simulink model "Identyfikacja"  (R2015a)
settings: Solver=ode4  StartTime=0.0  StopTime=tSim  FixedStep=0.01  RelTol=1e-3
values from neighbouring files (symbols this model uses):
  c1 = Parametry(1)    [skryptDoIdentyfikacji.m]    (also in wskaznikJakosci.m = params(1))
  c2 = Parametry(2)    [skryptDoIdentyfikacji.m]    (also in wskaznikJakosci.m = params(2))
  c3 = Parametry(3)    [skryptDoIdentyfikacji.m]    (also in wskaznikJakosci.m = params(3))
  p1 = polyfit(PWM_level, pred_napelniania, 2)    [chka_zawor_gora.m]    (also in skryptDoIdentyfikacji.m = [-49.142857142857010 99.114285714285490 -23.369999999999905]; wskaznikJakosci.m = [-49.142857142857010 99.114285714285490 -23.369999999999905])
  PWM = 0.4    [chka_zawor_gora.m]    (also in skryptDoIdentyfikacji.m = 1; wskaznikJakosci.m = 1)
settings Model: Creator=Kamil  LastModifiedBy=konra

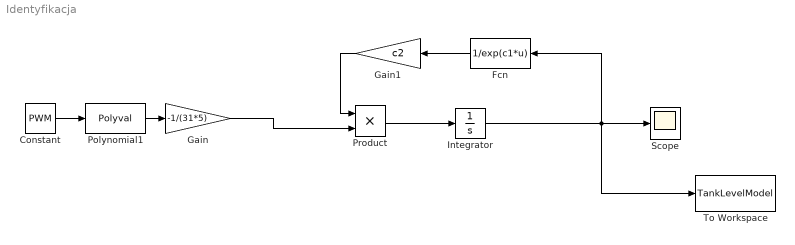
== system Identyfikacja ==
  Constant : Constant  Value=PWM
  Fcn : Fcn  Expr=1/exp(c1*u)
  Gain : Gain  Gain=-1/(31*5)
  Gain1 : Gain  Gain=c2
  Integrator : Integrator  InitialCondition=c3
  Polynomial1 : Polyval  Coefs=p1
  Product : Product
  Scope : Scope
      settings: TimeRange=180
  To Workspace : ToWorkspace  VariableName=TankLevelModel  SaveFormat=Structure With Time  SampleTime=-1
  wires:
  Integrator/1 -> Scope/1, To Workspace/1, Fcn/1
  Gain/1 -> Product/2
  Product/1 -> Integrator/1
  Fcn/1 -> Gain1/1
  Gain1/1 -> Product/1
  Constant/1 -> Polynomial1/1
  Polynomial1/1 -> Gain/1
